simulink model "Control_Flow"  (R2024b)
settings: Solver=VariableStepAuto  StartTime=0.0  StopTime=360.0  RelTol=1e-8
values from neighbouring files (symbols this model uses):
  kD = 1    [Aero560Project.m]
  kD_g = 1    [Aero560Project.m]
  kP = 0.1    [Aero560Project.m]
  kP_g = 0.1    [Aero560Project.m]
  omega0_42 = [alphaS0dot_42;betaS0dot_42;gammaS0dot_42]    [Aero560Project.m]
  Omega_SP = [0; 0; omegaSP]    [Aero560Project.m]
  quat0_42 = [quat0_42a(2); quat0_42a(3); quat0_42a(4); quat0_42a(1)]    [Aero560Project.m]
  targetAngles_42 = [alphaTgt_42;betaTgt_42;gammaTgt_42]    [Aero560Project.m]
  thetaG_42 = deg2rad(12.3)    [Aero560Project.m]
  thetaG_init = deg2rad(60)    [Aero560Project.m]
undefined symbols (not defined in the file or in its folder): params
libraries: sharedtransform x2, simulink_extras x1
settings Model: Creator=paigejewell  LastModifiedBy=bedag

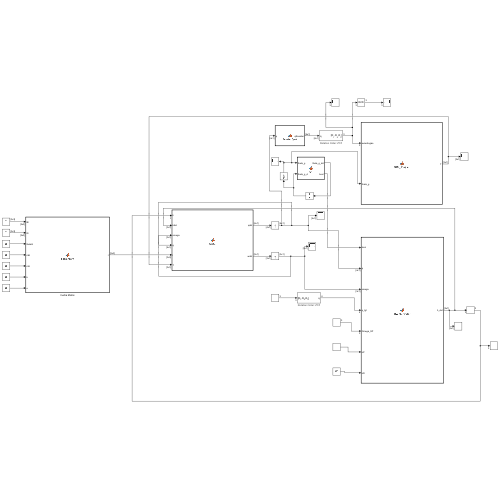
[thumbnail: Simulink's stored preview of the top-level diagram]
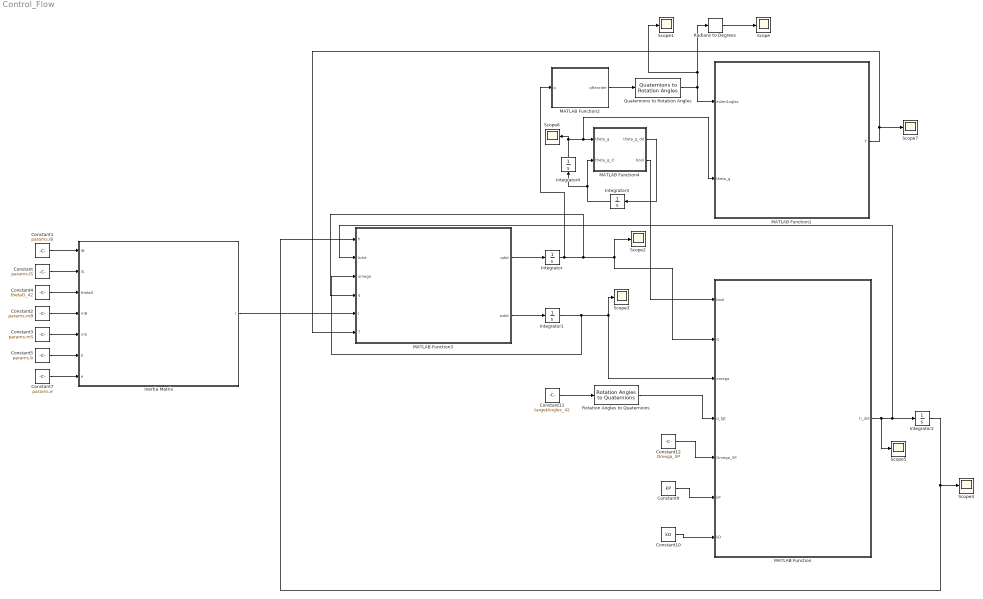
== system Control_Flow ==
  Constant : Constant  Value=params.IS
  Constant1 : Constant  Value=params.IB
  Constant10 : Constant  Value=kD
  Constant11 : Constant  Value=targetAngles_42
  Constant12 : Constant  Value=Omega_SP
  Constant2 : Constant  Value=params.mB
  Constant3 : Constant  Value=params.mS
  Constant4 : Constant  Value=thetaG_42
  Constant5 : Constant  Value=params.b
  Constant7 : Constant  Value=params.e
  Constant9 : Constant  Value=kP
  Inertia Matrix : MATLAB Function  TreatAsAtomicUnit=on
  Integrator : Integrator  InitialCondition=quat0_42
  Integrator1 : Integrator  InitialCondition=omega0_42
  Integrator2 : Integrator  InitialCondition=[0;0;0]
  Integrator3 : Integrator
  Integrator4 : Integrator  InitialCondition=thetaG_init
  MATLAB Function : MATLAB Function  TreatAsAtomicUnit=on
  MATLAB Function1 : MATLAB Function  TreatAsAtomicUnit=on
  MATLAB Function2 : MATLAB Function  TreatAsAtomicUnit=on
  MATLAB Function3 : MATLAB Function  TreatAsAtomicUnit=on
  MATLAB Function4 : MATLAB Function  TreatAsAtomicUnit=on
  Quaternions to Rotation Angles : sharedtransform/Quaternions to Rotation Angles  rotationOrder=ZYZ  aMode=aMode
  Radians to Degrees : simulink_extras/Transformations/Radians to Degrees
  Rotation Angles to Quaternions : sharedtransform/Rotation Angles to Quaternions  rotationOrder=ZYZ  aMode=aMode
  Scope{,1..7} (8 alike) : Scope
  wires:
  Constant/1 -> Inertia Matrix/2(IS)
  Constant1/1 -> Inertia Matrix/1(IB)
  Constant2/1 -> Inertia Matrix/4(mB)
  Constant3/1 -> Inertia Matrix/5(mS)
  Constant5/1 -> Inertia Matrix/6(b)
  Constant7/1 -> Inertia Matrix/7(e)
  Constant4/1 -> Inertia Matrix/3(thetaG)
  Quaternions to Rotation Angles/1 -> MATLAB Function1/1(eulerAngles), Scope1/1, Radians to Degrees/1
  MATLAB Function2/1(qReorder) -> Quaternions to Rotation Angles/1
  Constant9/1 -> MATLAB Function/6(kP)
  Constant10/1 -> MATLAB Function/7(kD)
  Inertia Matrix/1(I) -> MATLAB Function3/5(I)
  MATLAB Function3/1(qdot) -> Integrator/1
  MATLAB Function3/2(wdot) -> Integrator1/1
  Integrator/1 -> MATLAB Function3/4(q), Scope2/1, MATLAB Function/2(q), MATLAB Function2/1(q)
  Integrator1/1 -> MATLAB Function3/3(omega), Scope3/1, MATLAB Function/3(omega)
  MATLAB Function/1(h_dot) -> MATLAB Function3/2(hdot), Integrator2/1, Scope5/1
  Integrator2/1 -> Scope4/1, MATLAB Function3/1(h)
  MATLAB Function1/1(T) -> MATLAB Function3/6(T), Scope7/1
  Rotation Angles to Quaternions/1 -> MATLAB Function/4(q_tgt)
  Constant11/1 -> Rotation Angles to Quaternions/1
  Constant12/1 -> MATLAB Function/5(Omega_SP)
  Radians to Degrees/1 -> Scope/1
  MATLAB Function4/1(theta_g_dd) -> Integrator3/1
  Integrator3/1 -> Integrator4/1, MATLAB Function4/2(theta_g_d)
  MATLAB Function4/2(bool) -> MATLAB Function/1(bool)
  Integrator4/1 -> Scope6/1, MATLAB Function1/2(theta_g), MATLAB Function4/1(theta_g)

== matlab function Control_Flow/MATLAB Function ==
  data: bool input; q input; h_dot output; omega input; q_tgt input; Omega_SP input; kP input; kD input
function h_dot = RW_Controller(bool, q, omega, q_tgt, Omega_SP, kP, kD)
 
% Reorder Quaternion
q_current = [q(1);q(2);q(3);q(4)];

% Reorder Quaternion
q_c = [q_tgt(2);q_tgt(3);q_tgt(4);q_tgt(1)];

big_matrix = [ q_c(4) q_c(3) -q_c(2) -q_c(1);
               -q_c(3) q_c(4) q_c(1) -q_c(2);
               q_c(2) -q_c(1) q_c(4) -q_c(3);
               q_c(1) q_c(2)  q_c(3)  q_c(4)];

% Convert normalized quaternion to Wie convention
q_err = big_matrix * q_current;
% q_error_trunc = [q_error(1) q_error(2) q_error(3)]';

% Compute error quaternion (q_tgt^-1 * q_current)
% q_err = quat_multiply(quat_inv(q_tgt), q);

% q_bar_e is the vector part (Eq 39)
q_bar_e = q_err(1:3) * sign(q_err(4));

% Proportional term (Eq 39)
h_dot_P = kP * q_bar_e;

% Derivative term (Eq 39)  
% Omega_SP = [0; 0; Omega] for circular orbit
h_dot_D = kD * (omega - Omega_SP);

if bool == true
    h_dot = h_dot_P + h_dot_D;
    if h_dot == zeros(3,1)
        bool = false;
    end
else
    h_dot = zeros(3,1);
end
end

== matlab function Control_Flow/Inertia Matrix ==
  data: IB input; I output; IS input; thetaG input; mB input; mS input; b input; e input
function I = InertiaMatrix(IB, IS, thetaG, mB, mS, b, e)

c = cos(thetaG);
s = sin(thetaG);
M = mB + mS;

% Rotate I_B from body frame into sail frame
RotY = [c, 0, s; 0, 1, 0; -s, 0, c];
IB_SailFrame = RotY * IB * RotY';

% Offsets of each CoM from the system CoM
rhoB = [-b*s * mS/M;
         0;
         mS*(b*c + e)/M];

rhoS = [mB*b*s/M;
        0;
        -mB*(b*c + e)/M];

% Parallel axis theorem
DeltaB = mB * (dot(rhoB, rhoB)*eye(3) - rhoB*rhoB');
DeltaS = mS * (dot(rhoS, rhoS)*eye(3) - rhoS*rhoS');

% Total inertia matrix in sail frame
I = IB_SailFrame + IS + DeltaB + DeltaS;

end

== matlab function Control_Flow/MATLAB Function1 ==
  data: eulerAngles input; T output; theta_g input; params parameter
function T = SRP_Torque(eulerAngles,theta_g, params)

Theta_i = params.thetai;
a = params.a;
b = params.b;
d = params.d;
e = params.e;
Ca = params.Ca;
Cs = params.Cs;
Cd = params.Cd;
Bf = params.Bf;
P = params.P;
Ap = params.Ap;
mb = params.mB;
ms = params.mS;

% Compute xt, zt
xt = b*mb*sin(theta_g)/(mb+ms);
zt = (b*mb*cos(theta_g) + d*mb + (d-e)*ms)/(mb+ms);

% alpha = eulerAngles(1);
beta = eulerAngles(2);
gamma = eulerAngles(3);

l = a/(3*cos(Theta_i));

% Torque Equations in the Sail Frame
% Eq (16) - TxS
TxS = 2*P*Ap*zt*cos(Theta_i)*sin(beta)*sin(gamma) * ...
      (2*(Ca + 2*Cs*sin(Theta_i)^2 + Cd)*cos(beta) + ...
       Bf*Cd*sin(Theta_i)*tan(Theta_i)) ...
    - 2*P*Ap*l*sin(Theta_i)*sin(beta)*sin(gamma) * ...
      ((3*Ca + 4*Cs + 3*Cd)*cos(Theta_i)*cos(beta) + Bf*Cd);

% Eq (17) - TyS
TyS = 4*P*Ap*xt*cos(Theta_i)*((Ca + Cs*(-3*sin(Theta_i)^2 + 2) + Cd)* ...
    cos(beta)^2 + Bf*Cd*cos(Theta_i)*cos(beta) + Cs*sin(Theta_i)^2) + ...
    2*P*Ap*zt*cos(Theta_i)*sin(beta)*cos(gamma)*(2*(Ca + 2*Cs*sin(Theta_i)^2 + ...
    Cd)*cos(beta) + Bf*Cd*sin(Theta_i)*tan(Theta_i)) - 2*P*Ap*l*sin(Theta_i)* ...
    sin(beta)*cos(gamma)*((3*Ca + 4*Cs + 3*Cd)*cos(Theta_i)*cos(beta) + Bf*Cd);

% Eq (18) - TzS
TzS = 2*P*Ap*xt*sin(beta)*sin(gamma)*(-2*(Ca + 2*Cs*sin(Theta_i)^2 + Cd)*...
    cos(Theta_i)*cos(beta) - Bf*Cd*sin(Theta_i)^2);

T = [TxS; TyS; TzS];
end

== matlab function Control_Flow/MATLAB Function2 ==
  data: q input; qReorder output
function qReorder = ReorderQuat(q)

qReorder = [q(4);q(1);q(2);q(3)];

end

== matlab function Control_Flow/MATLAB Function3 ==
  data: qdot output size=[4 1]; h input; hdot input; omega input; q input; wdot output size=[3 1]; I input; T input
function [qdot,wdot] = State(h,hdot,omega,q,I,T)

epsilon = [q(1) q(2) q(3)]';
eta = q(4);
wcross = [0,-omega(3),omega(2);omega(3),0,-omega(1);-omega(2),omega(1),0];

wdot = I\(T - hdot - wcross*(I*omega+h));

ecross = [0,-epsilon(3),epsilon(2);epsilon(3),0,-epsilon(1);-epsilon(2),epsilon(1),0];

deps = 0.5*(eta*eye(3)+ecross)*omega;
deta = -0.5*epsilon'*omega;
qdot = [deps; deta];

end

== matlab function Control_Flow/MATLAB Function4 ==
  data: theta_g input; theta_g_d input; theta_g_dd output; kP_g parameter; kD_g parameter; thetaG_42 parameter; bool output
function [theta_g_dd, bool] = fcn(theta_g, theta_g_d, kP_g, kD_g, thetaG_42)

bool = false;

e = theta_g-thetaG_42;

theta_g_dd = -kP_g*e - kD_g*theta_g_d;

if abs(e)<0.01
    bool = true;
end

end
